simulink model "SF031A_CurrReasbnDiagc"  (R2013b)
settings: Solver=FixedStepDiscrete  SolverMode=SingleTasking  StartTime=0.0  StopTime=1  FixedStep=0.000125  RelTol=1e-3
values from neighbouring files (symbols this model uses):
  ARCHGLBPRM_2MILLISEC_SEC_F32 = DataDict.Constant    [SF031A_CurrReasbnDiagc_DataDict.m]
  ARCHGLBPRM_2PI_ULS_F32 = DataDict.Constant    [SF031A_CurrReasbnDiagc_DataDict.m]
  CurrReasbnDiagcCurrDiagcMotEnvlpTblMax = DataDict.Calibration    [SF031A_CurrReasbnDiagc_DataDict.m]
  CurrReasbnDiagcCurrDiagcPrimErrThd = DataDict.Calibration    [SF031A_CurrReasbnDiagc_DataDict.m]
  CurrReasbnDiagcCurrDiagcSecdryErrThd = DataDict.Calibration    [SF031A_CurrReasbnDiagc_DataDict.m]
  CurrReasbnDiagcCurrDiagcSecdryTqLimThd = DataDict.Calibration    [SF031A_CurrReasbnDiagc_DataDict.m]
  CurrReasbnDiagcDiagFildLim = DataDict.Calibration    [SF031A_CurrReasbnDiagc_DataDict.m]
  CurrReasbnDiagcDiagVltgLpFilEna = DataDict.Calibration    [SF031A_CurrReasbnDiagc_DataDict.m]
  CurrReasbnDiagcLpFilSca = DataDict.Calibration    [SF031A_CurrReasbnDiagc_DataDict.m]
  CurrReasbnDiagcMotVelHiLim = DataDict.Calibration    [SF031A_CurrReasbnDiagc_DataDict.m]
  CurrReasbnDiagcMotVelLoLim = DataDict.Calibration    [SF031A_CurrReasbnDiagc_DataDict.m]
  CurrReasbnDiagcMotVltgQaxDaxFilEna = DataDict.Calibration    [SF031A_CurrReasbnDiagc_DataDict.m]
  CurrReasbnDiagcVelLpFilEna = DataDict.Calibration    [SF031A_CurrReasbnDiagc_DataDict.m]
  ELECGLBPRM_PWMPERDNOMX2_SEC_F32 = DataDict.ConfigParam    [SF031A_CurrReasbnDiagc_DataDict.m]
  NODEBSTEP_CNT_U16 = DataDict.Constant    [SF031A_CurrReasbnDiagc_DataDict.m]
  OffsErrExcdd = DataDict.NTC    [SF031A_CurrReasbnDiagc_DataDict.m]
  ONE_ULS_F32 = DataDict.Constant    [SF031A_CurrReasbnDiagc_DataDict.m]
  ONEOVERTWO_ULS_F32 = DataDict.Constant    [SF031A_CurrReasbnDiagc_DataDict.m]
  SysGlbPrmMotPoleCnt = DataDict.ImprtdCal    [SF031A_CurrReasbnDiagc_DataDict.m]
  TWO_ULS_F32 = DataDict.Constant    [SF031A_CurrReasbnDiagc_DataDict.m]
undefined symbols (not defined in the file or in its folder): NtcSts1
libraries: Fil x8, simulink x6, NxtrLim x3, NxtrMath x2, NexteerUtilities x1
(part 1 of 2)
settings Model: Creator=SZJ6LD  LastModifiedBy=XZ3VZ1
settings DataIOCC: SaveFormat=Structure
settings DebuggingCC: UnderspecifiedInitializationDetection=Simplified  MultiTaskDSMMsg=none

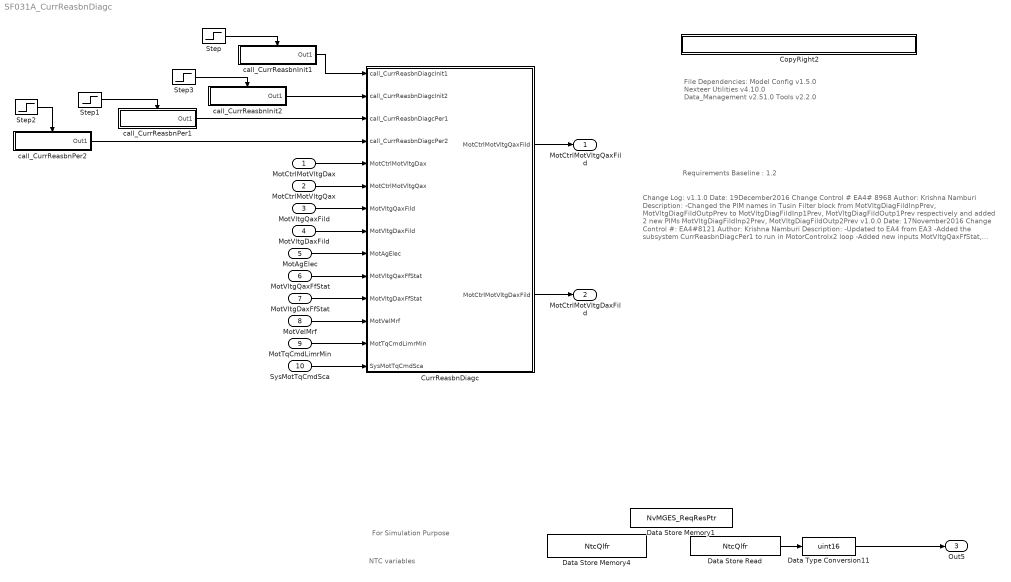
== system SF031A_CurrReasbnDiagc ==
  note: Requirements Baseline : 1.2
  note: File Dependencies:
      |
      | Model Config v1.5.0
      | Nexteer Utilities v4.10.0
      | Data_Management v2.51.0
      | Tools v2.2.0
  note: Change Log:
      |
      | v1.1.0
      | Date: 19December2016
      | Change Control # EA4# 8968
      | Author: Krishna Namburi
      | Description:
      | -Changed the PIM names in Tusin Filter block from MotVltgDiagFildInpPrev, MotVltgDiagFildOutpPrev
      | to  MotVltgDiagFildInp1Prev, MotVltgDiagFildOutp1Prev respectively and added 2 new PIMs
      | MotVltgDiagFildInp2Prev, MotVltgDiagFildOutp2Prev
      |
      | v1.0.0
      | Date: 17November2016
      | Change Control #: EA4#8121
      | Author: Krishna Namburi
      | Description:
      | -Updated to EA4 from EA3
      | -Added the subsystem CurrReasbnDiagcPer1 to run in MotorControlx2 loop
      | -Added new inputs MotVltgQaxFfStat, MotVltgDaxFfStat.
      | - Removed inputs MtrCurrQaxFinalRef_Amp_f32, MtrCurrDaxRef_Amp_f32,EstKe_VpRadpS_f32
      | EstR_Ohm_f32.
      | -Added new outputs MotCtrlMotVltgQaxFild and MotCtrlMotVltgDaxFild.
      | -Removed outputs MotCurrIdptSig_Cnt_u08
      | -Modified CurrReasbnDiagcPer2 subsystem and CurrReasbn Diagnostic subsystem
  note: For Simulation Purpose
  note: NTC variables
  MotCtrlMotVltgDax : Inport  RequirementInfo={} %GIDa_4d26a9da_0edf_44cc_96b7_6099ab8f4765
  MotCtrlMotVltgQax : Inport  RequirementInfo={} %GIDa_b123e9bc_32a7_4223_a27c_0bbcef9fd6da  Port=2
  MotVltgQaxFild : Inport  RequirementInfo={} %GIDa_1c53ad45_08f1_44a0_80ec_49126e27887e  Port=3
  MotVltgDaxFild : Inport  RequirementInfo={} %GIDa_c9186f2c_0f7b_428f_a1bb_4953a8fb6071  Port=4
  MotAgElec : Inport  RequirementInfo={} %GIDa_1a6fc1e2_263f_4c35_82dc_8d7ad84c14ca  Port=5
  MotVltgQaxFfStat : Inport  RequirementInfo={} %GIDa_f597cf15_84d9_42b9_a8ac_86a604ca58ec  Port=6
  MotVltgDaxFfStat : Inport  RequirementInfo={} %GIDa_437fa6bb_7f66_4ed8_b004_d7df1d456be5  Port=7
  MotVelMrf : Inport  RequirementInfo={} %GIDa_277e3cf7_0a4f_44b2_8f78_f4d7dd669071  Port=8
  MotTqCmdLimrMin : Inport  RequirementInfo={} %GIDa_9d945749_2d47_417b_b7b0_0809e9f72747  Port=9
  SysMotTqCmdSca : Inport  RequirementInfo={} %GIDa_449e895f_222c_4d81_855c_0e9bc98e4ae6  Port=10
  CopyRight2 : Subsystem  Description=|  mask(Copyright Information){none=on}
      | Copyright info block.                                               
      |                                                                     
      | Place copyright information at the top of every subsystem in design.
      mask prompts: none "No parameters"
      mask help: Place copyright information at the top of every subsystem in design.
      mask Display:
      | NxtrConf = 'Nexteer Confidential';
      | 
      | sys = bdroot; %handle for the current model ("system")
      | first = get_param(sys,'Created');
      | if(isempty(first))
      |     first = datestr(now,'yyyy');
      | else
      |     first = first(end-3:end);  %year is last four digits
      | end
      | 
      | last = get_param(sys,'LastModifiedDate');
      | if isempty(last)
      |     last = datestr(now,'yyyy');
      | else
      |     last = last(end-3:end);
      | end
      | 
      | if strcmp(first,last)
      |     fprintf('%s -- Copyright %s Nexteer',NxtrConf,first)
      | else
      |     fprintf('%s -- %s%s- %s Nexteer',NxtrConf,char(169),first,last)
      | end
  CurrReasbnDiagc : Subsystem
  Data Store Memory1 : DataStoreMemory  DataStoreName=NvMGES_ReqResPtr  OutDataTypeStr=uint8
  Data Store Read : DataStoreRead  DataStoreName=NtcQlfr  SampleTime=0.1
  Data Store Memory4 : DataStoreMemory  DataStoreName=NtcQlfr  InitialValue=SigQlfr1.SIGQLFR_NORES  OutDataTypeStr=Enum: SigQlfr1
  Data Type Conversion11 : DataTypeConversion  OutDataTypeStr=uint16
  Step : Step  Before=1  After=0  SampleTime=0.000125
  Step1 : Step  SampleTime=0.000125
  Step2 : Step  SampleTime=0.002
  Step3 : Step  Before=1  After=0  SampleTime=0.002
  call_CurrReasbnInit1 : Subsystem  TreatAsAtomicUnit=on
  call_CurrReasbnInit2 : Subsystem  TreatAsAtomicUnit=on
  call_CurrReasbnPer1 : Subsystem  TreatAsAtomicUnit=on
  call_CurrReasbnPer2 : Subsystem  TreatAsAtomicUnit=on
  MotCtrlMotVltgQaxFild : Outport
  MotCtrlMotVltgDaxFild : Outport  Port=2
  Out5 : Outport  Port=3
  wires:
  MotCtrlMotVltgDax/1 -> CurrReasbnDiagc/5(MotCtrlMotVltgDax)
  MotVelMrf/1 -> CurrReasbnDiagc/12(MotVelMrf)
  MotTqCmdLimrMin/1 -> CurrReasbnDiagc/13(MotTqCmdLimrMin)
  SysMotTqCmdSca/1 -> CurrReasbnDiagc/14(SysMotTqCmdSca)
  call_CurrReasbnPer2/1(Out1) -> CurrReasbnDiagc/4(call_CurrReasbnDiagcPer2)
  Step/1 -> call_CurrReasbnInit1/Enable
  Step2/1 -> call_CurrReasbnPer2/Enable
  call_CurrReasbnInit1/1(Out1) -> CurrReasbnDiagc/1(call_CurrReasbnDiagcInit1)
  call_CurrReasbnPer1/1(Out1) -> CurrReasbnDiagc/3(call_CurrReasbnDiagcPer1)
  MotVltgDaxFfStat/1 -> CurrReasbnDiagc/11(MotVltgDaxFfStat)
  MotVltgQaxFfStat/1 -> CurrReasbnDiagc/10(MotVltgQaxFfStat)
  MotAgElec/1 -> CurrReasbnDiagc/9(MotAgElec)
  MotCtrlMotVltgQax/1 -> CurrReasbnDiagc/6(MotCtrlMotVltgQax)
  MotVltgQaxFild/1 -> CurrReasbnDiagc/7(MotVltgQaxFild)
  MotVltgDaxFild/1 -> CurrReasbnDiagc/8(MotVltgDaxFild)
  Step1/1 -> call_CurrReasbnPer1/Enable
  CurrReasbnDiagc/1(MotCtrlMotVltgQaxFild) -> MotCtrlMotVltgQaxFild/1
  CurrReasbnDiagc/2(MotCtrlMotVltgDaxFild) -> MotCtrlMotVltgDaxFild/1
  Data Store Read/1 -> Data Type Conversion11/1
  Data Type Conversion11/1 -> Out5/1
  Step3/1 -> call_CurrReasbnInit2/Enable
  call_CurrReasbnInit2/1(Out1) -> CurrReasbnDiagc/2(call_CurrReasbnDiagcInit2)

== system SF031A_CurrReasbnDiagc/CopyRight2 ==

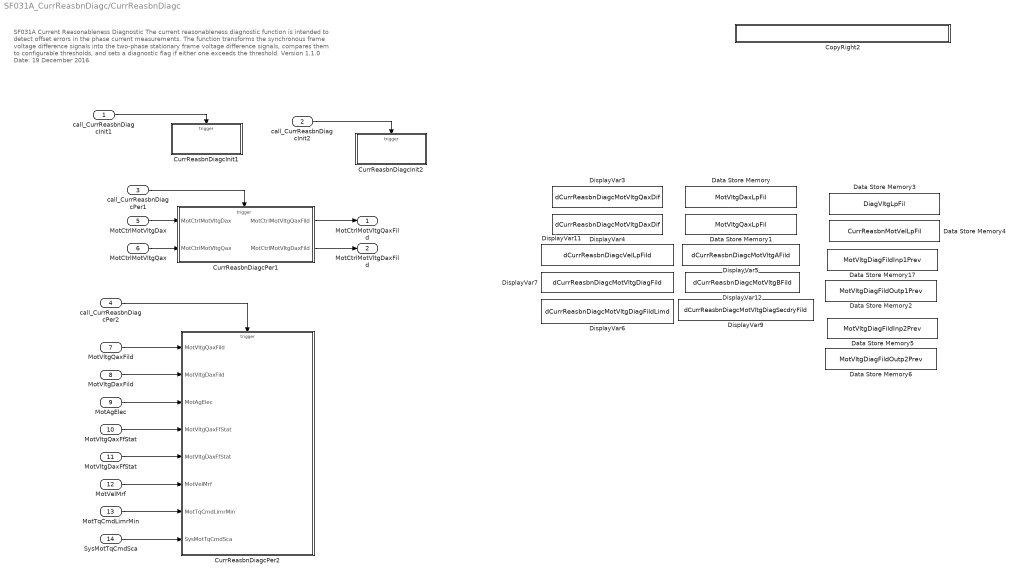
== system SF031A_CurrReasbnDiagc/CurrReasbnDiagc ==
  note: SF031A Current Reasonableness Diagnostic
      |
      | The current reasonableness diagnostic function is intended to detect offset errors in the phase current measurements.
      | The function transforms the synchronous frame voltage difference signals into the two-phase stationary frame voltage difference signals,
      | compares them to configurable thresholds, and sets a diagnostic flag if either one exceeds the threshold.
      | Version 1.1.0   						Date: 19 December 2016
  call_CurrReasbnDiagcInit1 : Inport
  call_CurrReasbnDiagcInit2 : Inport  Port=2
  call_CurrReasbnDiagcPer1 : Inport  RequirementInfo={} %GIDa_f76a18cf_877e_4c65_9912_3a0b33b85457  Port=3
  call_CurrReasbnDiagcPer2 : Inport  RequirementInfo={} %GIDa_cd620524_5019_4baf_8954_3888c8ee52e6  Port=4
  MotCtrlMotVltgDax : Inport  RequirementInfo="{'linktype_rmi_doors' '0000a538 (/E-STEER Core/SubSystem Specifications/Application Functions/SF031A Current Reasonableness Diagnostic)' '#SF031A_101' 'true' 'REQ:  SF031A_101' '' } %GIDa_449d6a4b_7542_48a4_994b_5c51cb8953a2"  Port=5
  MotCtrlMotVltgQax : Inport  RequirementInfo="{'linktype_rmi_doors' '0000a538 (/E-STEER Core/SubSystem Specifications/Application Functions/SF031A Current Reasonableness Diagnostic)' '#SF031A_102' 'true' 'REQ:  SF031A_102' '' } %GIDa_a31c9886_c939_4f41_ac5c_04f44dc75ab9"  Port=6
  MotVltgQaxFild : Inport  RequirementInfo="{'linktype_rmi_doors' '0000a538 (/E-STEER Core/SubSystem Specifications/Application Functions/SF031A Current Reasonableness Diagnostic)' '#SF031A_180' 'true' 'REQ:  SF031A_180' '' } %GIDa_58e0e7bc_af85_4941_a339_39c564b14f0e"  Port=7
  MotVltgDaxFild : Inport  RequirementInfo="{'linktype_rmi_doors' '0000a538 (/E-STEER Core/SubSystem Specifications/Application Functions/SF031A Current Reasonableness Diagnostic)' '#SF031A_181' 'true' 'REQ:  SF031A_181' '' } %GIDa_79f235f9_d307_415b_b321_c5cb8a8df617"  Port=8
  MotAgElec : Inport  RequirementInfo="{'linktype_rmi_doors' '0000a538 (/E-STEER Core/SubSystem Specifications/Application Functions/SF031A Current Reasonableness Diagnostic)' '#SF031A_105' 'true' 'REQ:  SF031A_105' '' } %GIDa_d9cd6df8_3f02_4782_98d1_16055f3fe8b2"  Port=9
  MotVltgQaxFfStat : Inport  RequirementInfo="{'linktype_rmi_doors' '0000a538 (/E-STEER Core/SubSystem Specifications/Application Functions/SF031A Current Reasonableness Diagnostic)' '#SF031A_104' 'true' 'REQ:  SF031A_104' '' } %GIDa_abd8e3fa_7b87_4c29_ad4d_b706a14441a8"  Port=10
  MotVltgDaxFfStat : Inport  RequirementInfo="{'linktype_rmi_doors' '0000a538 (/E-STEER Core/SubSystem Specifications/Application Functions/SF031A Current Reasonableness Diagnostic)' '#SF031A_103' 'true' 'REQ:  SF031A_103' '' } %GIDa_fd47e6d3_2ce2_43f3_87fa_49b3cc0c72b9"  Port=11
  MotVelMrf : Inport  RequirementInfo="{'linktype_rmi_doors' '0000a538 (/E-STEER Core/SubSystem Specifications/Application Functions/SF031A Current Reasonableness Diagnostic)' '#SF031A_113' 'true' 'REQ:  SF031A_113' '' } %GIDa_c5440ddd_8457_4693_9dbb_e70183087e81"  Port=12
  MotTqCmdLimrMin : Inport  RequirementInfo="{'linktype_rmi_doors' '0000a538 (/E-STEER Core/SubSystem Specifications/Application Functions/SF031A Current Reasonableness Diagnostic)' '#SF031A_34' 'true' 'REQ:  SF031A_34' '' } %GIDa_c2343a4c_6c51_4dbf_8cb4_7c8b57a50bd8"  Port=13
  SysMotTqCmdSca : Inport  RequirementInfo="{'linktype_rmi_doors' '0000a538 (/E-STEER Core/SubSystem Specifications/Application Functions/SF031A Current Reasonableness Diagnostic)' '#SF031A_32' 'true' 'REQ:  SF031A_32' '' } %GIDa_aa36bb47_abbb_4a1b_9669_fdecfc6ed391"  Port=14
  CopyRight2 : Subsystem  Description=|  mask(Copyright Information){none=on}
      | Copyright info block.                                               
      |                                                                     
      | Place copyright information at the top of every subsystem in design.
      mask prompts: none "No parameters"
      mask help: Place copyright information at the top of every subsystem in design.
      mask Display:
      | NxtrConf = 'Nexteer Confidential';
      | 
      | sys = bdroot; %handle for the current model ("system")
      | first = get_param(sys,'Created');
      | if(isempty(first))
      |     first = datestr(now,'yyyy');
      | else
      |     first = first(end-3:end);  %year is last four digits
      | end
      | 
      | last = get_param(sys,'LastModifiedDate');
      | if isempty(last)
      |     last = datestr(now,'yyyy');
      | else
      |     last = last(end-3:end);
      | end
      | 
      | if strcmp(first,last)
      |     fprintf('%s -- Copyright %s Nexteer',NxtrConf,first)
      | else
      |     fprintf('%s -- %s%s- %s Nexteer',NxtrConf,char(169),first,last)
      | end
  CurrReasbnDiagcInit1 : Subsystem
  CurrReasbnDiagcInit2 : Subsystem
  CurrReasbnDiagcPer1 : Subsystem
  CurrReasbnDiagcPer2 : Subsystem
  Data Store Memory : DataStoreMemory  DataStoreName=MotVltgDaxLpFil  InitialValue=[]  StateMustResolveToSignalObject=on
  Data Store Memory1 : DataStoreMemory  DataStoreName=MotVltgQaxLpFil  InitialValue=[]  StateMustResolveToSignalObject=on
  Data Store Memory17 : DataStoreMemory  DataStoreName=MotVltgDiagFildInp1Prev  StateMustResolveToSignalObject=on
  Data Store Memory2 : DataStoreMemory  DataStoreName=MotVltgDiagFildOutp1Prev  StateMustResolveToSignalObject=on
  Data Store Memory3 : DataStoreMemory  DataStoreName=DiagVltgLpFil  InitialValue=[]  StateMustResolveToSignalObject=on
  Data Store Memory4 : DataStoreMemory  DataStoreName=CurrReasbnMotVelLpFil  InitialValue=[]  StateMustResolveToSignalObject=on
  Data Store Memory5 : DataStoreMemory  DataStoreName=MotVltgDiagFildInp2Prev  StateMustResolveToSignalObject=on
  Data Store Memory6 : DataStoreMemory  DataStoreName=MotVltgDiagFildOutp2Prev  StateMustResolveToSignalObject=on
  DisplayVar11 : DataStoreMemory  DataStoreName=dCurrReasbnDiagcVelLpFild  ReadBeforeWriteMsg=warning  WriteAfterWriteMsg=warning  WriteAfterReadMsg=warning  StateMustResolveToSignalObject=on
  DisplayVar12 : DataStoreMemory  DataStoreName=dCurrReasbnDiagcMotVltgBFild  ReadBeforeWriteMsg=warning  WriteAfterWriteMsg=warning  WriteAfterReadMsg=warning  StateMustResolveToSignalObject=on
  DisplayVar3 : DataStoreMemory  DataStoreName=dCurrReasbnDiagcMotVltgQaxDif  ReadBeforeWriteMsg=warning  WriteAfterWriteMsg=warning  WriteAfterReadMsg=warning  StateMustResolveToSignalObject=on
  DisplayVar4 : DataStoreMemory  DataStoreName=dCurrReasbnDiagcMotVltgDaxDif  ReadBeforeWriteMsg=warning  WriteAfterWriteMsg=warning  WriteAfterReadMsg=warning  StateMustResolveToSignalObject=on
  DisplayVar5 : DataStoreMemory  DataStoreName=dCurrReasbnDiagcMotVltgAFild  ReadBeforeWriteMsg=warning  WriteAfterWriteMsg=warning  WriteAfterReadMsg=warning  StateMustResolveToSignalObject=on
  DisplayVar6 : DataStoreMemory  DataStoreName=dCurrReasbnDiagcMotVltgDiagFildLimd  ReadBeforeWriteMsg=warning  WriteAfterWriteMsg=warning  WriteAfterReadMsg=warning  StateMustResolveToSignalObject=on
  DisplayVar7 : DataStoreMemory  DataStoreName=dCurrReasbnDiagcMotVltgDiagFild  ReadBeforeWriteMsg=warning  WriteAfterWriteMsg=warning  WriteAfterReadMsg=warning  StateMustResolveToSignalObject=on
  DisplayVar9 : DataStoreMemory  DataStoreName=dCurrReasbnDiagcMotVltgDiagSecdryFild  ReadBeforeWriteMsg=warning  WriteAfterWriteMsg=warning  WriteAfterReadMsg=warning  StateMustResolveToSignalObject=on
  MotCtrlMotVltgQaxFild : Outport  RequirementInfo="{'linktype_rmi_doors' '0000a538 (/E-STEER Core/SubSystem Specifications/Application Functions/SF031A Current Reasonableness Diagnostic)' '#SF031A_183' 'true' 'REQ:  SF031A_183' '' ; 'linktype_rmi_doors' '0000a538 (/E-STEER Core/SubSystem Specifications/Application Functions/SF031A Current Reasonableness Diagnostic)' '#SF031A_53' 'true' 'REQ:  SF031A_53' '' } %GIDa_ce180fd6_f185_48df_8933_7de0682d2221"
  MotCtrlMotVltgDaxFild : Outport  RequirementInfo="{'linktype_rmi_doors' '0000a538 (/E-STEER Core/SubSystem Specifications/Application Functions/SF031A Current Reasonableness Diagnostic)' '#SF031A_184' 'true' 'REQ:  SF031A_184' '' ; 'linktype_rmi_doors' '0000a538 (/E-STEER Core/SubSystem Specifications/Application Functions/SF031A Current Reasonableness Diagnostic)' '#SF031A_188' 'true' 'REQ:  SF031A_188' '' } %GIDa_5c3c9398_cb08_40a3_88f4_91205b1bad21"  Port=2
  wires:
  MotCtrlMotVltgDax/1 -> CurrReasbnDiagcPer1/1(MotCtrlMotVltgDax)
  MotCtrlMotVltgQax/1 -> CurrReasbnDiagcPer1/2(MotCtrlMotVltgQax)
  MotAgElec/1 -> CurrReasbnDiagcPer2/3(MotAgElec)
  MotVltgQaxFfStat/1 -> CurrReasbnDiagcPer2/4(MotVltgQaxFfStat)
  MotVltgDaxFfStat/1 -> CurrReasbnDiagcPer2/5(MotVltgDaxFfStat)
  MotVelMrf/1 -> CurrReasbnDiagcPer2/6(MotVelMrf)
  MotTqCmdLimrMin/1 -> CurrReasbnDiagcPer2/7(MotTqCmdLimrMin)
  SysMotTqCmdSca/1 -> CurrReasbnDiagcPer2/8(SysMotTqCmdSca)
  call_CurrReasbnDiagcInit1/1 -> CurrReasbnDiagcInit1/Trigger
  call_CurrReasbnDiagcPer1/1 -> CurrReasbnDiagcPer1/Trigger
  call_CurrReasbnDiagcPer2/1 -> CurrReasbnDiagcPer2/Trigger
  CurrReasbnDiagcPer1/1(MotCtrlMotVltgQaxFild) -> MotCtrlMotVltgQaxFild/1
  CurrReasbnDiagcPer1/2(MotCtrlMotVltgDaxFild) -> MotCtrlMotVltgDaxFild/1
  MotVltgQaxFild/1 -> CurrReasbnDiagcPer2/1(MotVltgQaxFild)
  MotVltgDaxFild/1 -> CurrReasbnDiagcPer2/2(MotVltgDaxFild)
  call_CurrReasbnDiagcInit2/1 -> CurrReasbnDiagcInit2/Trigger

== system SF031A_CurrReasbnDiagc/call_CurrReasbnInit1 ==
  Enable : EnablePort
  Function-Call Generator : simulink/Ports & Subsystems/Function-Call Generator  sample_time=0.000125  numberOfIterations=1
  Out1 : Outport
  wires:
  Function-Call Generator/1 -> Out1/1

== system SF031A_CurrReasbnDiagc/call_CurrReasbnInit2 ==
  Enable : EnablePort
  Function-Call Generator : simulink/Ports & Subsystems/Function-Call Generator  sample_time=0.002  numberOfIterations=1
  Out1 : Outport
  wires:
  Function-Call Generator/1 -> Out1/1

== system SF031A_CurrReasbnDiagc/call_CurrReasbnPer1 ==
  Enable : EnablePort
  Function-Call Generator : simulink/Ports & Subsystems/Function-Call Generator  sample_time=0.002  numberOfIterations=1
  Out1 : Outport
  wires:
  Function-Call Generator/1 -> Out1/1

== system SF031A_CurrReasbnDiagc/call_CurrReasbnPer2 ==
  Enable : EnablePort
  Function-Call Generator : simulink/Ports & Subsystems/Function-Call Generator  sample_time=0.1  numberOfIterations=1
  Out1 : Outport
  wires:
  Function-Call Generator/1 -> Out1/1

== system SF031A_CurrReasbnDiagc/CurrReasbnDiagc/CopyRight2 ==

== system SF031A_CurrReasbnDiagc/CurrReasbnDiagc/CurrReasbnDiagcInit1 ==
  Function : TriggerPort  TriggerType=function-call  PortDimensions=1
  CopyRight2 : Subsystem  Description=|  mask(Copyright Information){none=on}
      | Copyright info block.                                               
      |                                                                     
      | Place copyright information at the top of every subsystem in design.
      mask prompts: none "No parameters"
      mask help: Place copyright information at the top of every subsystem in design.
      mask Display:
      | NxtrConf = 'Nexteer Confidential';
      | 
      | sys = bdroot; %handle for the current model ("system")
      | first = get_param(sys,'Created');
      | if(isempty(first))
      |     first = datestr(now,'yyyy');
      | else
      |     first = first(end-3:end);  %year is last four digits
      | end
      | 
      | last = get_param(sys,'LastModifiedDate');
      | if isempty(last)
      |     last = datestr(now,'yyyy');
      | else
      |     last = last(end-3:end);
      | end
      | 
      | if strcmp(first,last)
      |     fprintf('%s -- Copyright %s Nexteer',NxtrConf,first)
      | else
      |     fprintf('%s -- %s%s- %s Nexteer',NxtrConf,char(169),first,last)
      | end
  MotVltgDaxLpFil : Fil/FilLpInit  RequirementInfo="{'linktype_rmi_doors' '0000a538 (/E-STEER Core/SubSystem Specifications/Application Functions/SF031A Current Reasonableness Diagnostic)' '#SF031A_117' 'true' 'REQ:  SF031A_117' '' ; 'linktype_rmi_doors' '0000a538 (/E-STEER Core/SubSystem Specifications/Application Functions/SF031A Current Reasonableness Diagnostic)' '#SF031A_118' 'true' 'REQ:  SF031A_118' '' ; 'linktype_rmi_doors' '0000a538 (/E-STEER Core/SubSystem Specifications/Application Functions/SF031A Current Reasonableness Diagnostic)' '#SF031A_119' 'true' 'REQ:  SF031A_119' '' } %GIDa_545bb3fc_f7bc_47c5_a864_b622a625ba7e"  Ic=0  Ts=ELECGLBPRM_PWMPERDNOMX2_SEC_F32  Freq=CurrReasbnDiagcMotVltgDaxLpFilFrq  StVar=MotVltgDaxLpFil
  MotVltgQaxLpFil : Fil/FilLpInit  RequirementInfo="{'linktype_rmi_doors' '0000a538 (/E-STEER Core/SubSystem Specifications/Application Functions/SF031A Current Reasonableness Diagnostic)' '#SF031A_120' 'true' 'REQ:  SF031A_120' '' ; 'linktype_rmi_doors' '0000a538 (/E-STEER Core/SubSystem Specifications/Application Functions/SF031A Current Reasonableness Diagnostic)' '#SF031A_121' 'true' 'REQ:  SF031A_121' '' ; 'linktype_rmi_doors' '0000a538 (/E-STEER Core/SubSystem Specifications/Application Functions/SF031A Current Reasonableness Diagnostic)' '#SF031A_122' 'true' 'REQ:  SF031A_122' '' } %GIDa_604bee18_9ac3_4a74_b746_90fd54a7749f"  Ic=0  Ts=ELECGLBPRM_PWMPERDNOMX2_SEC_F32  Freq=CurrReasbnDiagcMotVltgQaxLpFilFrq  StVar=MotVltgQaxLpFil

== system SF031A_CurrReasbnDiagc/CurrReasbnDiagc/CurrReasbnDiagcInit2 ==
  Function : TriggerPort  TriggerType=function-call  PortDimensions=1
  CopyRight2 : Subsystem  Description=|  mask(Copyright Information){none=on}
      | Copyright info block.                                               
      |                                                                     
      | Place copyright information at the top of every subsystem in design.
      mask prompts: none "No parameters"
      mask help: Place copyright information at the top of every subsystem in design.
      mask Display:
      | NxtrConf = 'Nexteer Confidential';
      | 
      | sys = bdroot; %handle for the current model ("system")
      | first = get_param(sys,'Created');
      | if(isempty(first))
      |     first = datestr(now,'yyyy');
      | else
      |     first = first(end-3:end);  %year is last four digits
      | end
      | 
      | last = get_param(sys,'LastModifiedDate');
      | if isempty(last)
      |     last = datestr(now,'yyyy');
      | else
      |     last = last(end-3:end);
      | end
      | 
      | if strcmp(first,last)
      |     fprintf('%s -- Copyright %s Nexteer',NxtrConf,first)
      | else
      |     fprintf('%s -- %s%s- %s Nexteer',NxtrConf,char(169),first,last)
      | end
  DiagVltgLpFil : Fil/FilLpInit  RequirementInfo="{'linktype_rmi_doors' '0000a538 (/E-STEER Core/SubSystem Specifications/Application Functions/SF031A Current Reasonableness Diagnostic)' '#SF031A_55' 'true' 'REQ:  SF031A_55' '' ; 'linktype_rmi_doors' '0000a538 (/E-STEER Core/SubSystem Specifications/Application Functions/SF031A Current Reasonableness Diagnostic)' '#SF031A_68' 'true' 'REQ:  SF031A_68' '' ; 'linktype_rmi_doors' '0000a538 (/E-STEER Core/SubSystem Specifications/Application Functions/SF031A Current Reasonableness Diagnostic)' '#SF031A_69' 'true' 'REQ:  SF031A_69' '' } %GIDa_a4e20848_ba57_4acb_8d1e_03c55eb94fa5"  Ic=0  Ts=ARCHGLBPRM_2MILLISEC_SEC_F32  Freq=CurrReasbnDiagcDiagVltgLpFilFrq  StVar=DiagVltgLpFil
  MotVelLpFil : Fil/FilLpInit  RequirementInfo="{'linktype_rmi_doors' '0000a538 (/E-STEER Core/SubSystem Specifications/Application Functions/SF031A Current Reasonableness Diagnostic)' '#SF031A_135' 'true' 'REQ:  SF031A_135' '' ; 'linktype_rmi_doors' '0000a538 (/E-STEER Core/SubSystem Specifications/Application Functions/SF031A Current Reasonableness Diagnostic)' '#SF031A_136' 'true' 'REQ:  SF031A_136' '' ; 'linktype_rmi_doors' '0000a538 (/E-STEER Core/SubSystem Specifications/Application Functions/SF031A Current Reasonableness Diagnostic)' '#SF031A_137' 'true' 'REQ:  SF031A_137' '' } %GIDa_38e4ad57_fc16_456c_8108_9d804f014d91"  Ic=0  Ts=ARCHGLBPRM_2MILLISEC_SEC_F32  Freq=CurrReasbnDiagcVelLpFilFrq  StVar=CurrReasbnMotVelLpFil

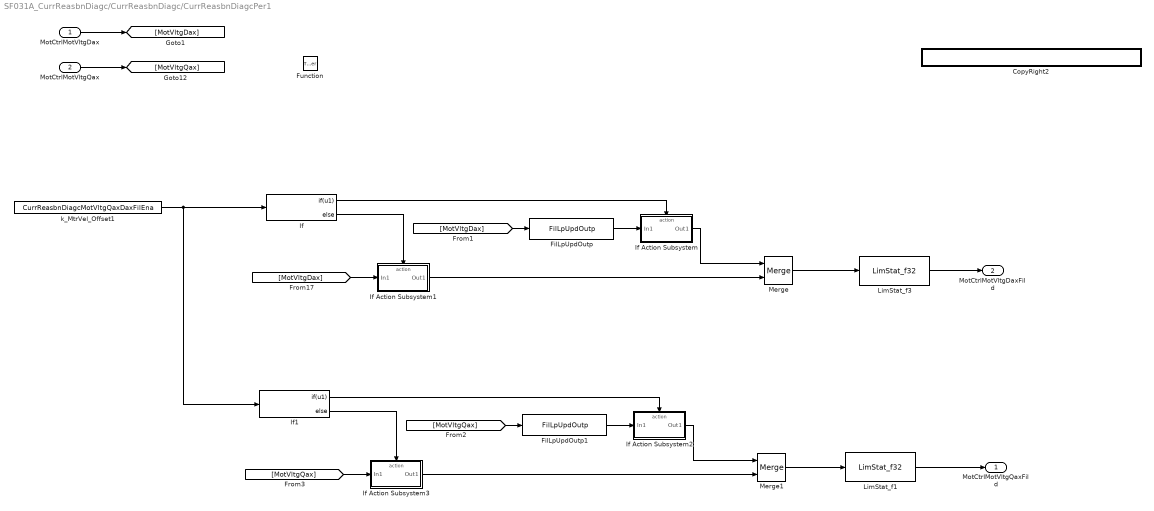
== system SF031A_CurrReasbnDiagc/CurrReasbnDiagc/CurrReasbnDiagcPer1 ==
  MotCtrlMotVltgDax : Inport
  MotCtrlMotVltgQax : Inport  Port=2
  Function : TriggerPort  TriggerType=function-call  PortDimensions=1
  CopyRight2 : Subsystem  Description=|  mask(Copyright Information){none=on}
      | Copyright info block.                                               
      |                                                                     
      | Place copyright information at the top of every subsystem in design.
      mask prompts: none "No parameters"
      mask help: Place copyright information at the top of every subsystem in design.
      mask Display:
      | NxtrConf = 'Nexteer Confidential';
      | 
      | sys = bdroot; %handle for the current model ("system")
      | first = get_param(sys,'Created');
      | if(isempty(first))
      |     first = datestr(now,'yyyy');
      | else
      |     first = first(end-3:end);  %year is last four digits
      | end
      | 
      | last = get_param(sys,'LastModifiedDate');
      | if isempty(last)
      |     last = datestr(now,'yyyy');
      | else
      |     last = last(end-3:end);
      | end
      | 
      | if strcmp(first,last)
      |     fprintf('%s -- Copyright %s Nexteer',NxtrConf,first)
      | else
      |     fprintf('%s -- %s%s- %s Nexteer',NxtrConf,char(169),first,last)
      | end
  FilLpUpdOutp : Fil/FilLpUpdOutp  RequirementInfo="{'linktype_rmi_doors' '0000a538 (/E-STEER Core/SubSystem Specifications/Application Functions/SF031A Current Reasonableness Diagnostic)' '#SF031A_119' 'true' 'REQ:  SF031A_119' '' } %GIDa_0bdcd772_3d94_4ed3_9d8e_9a962b62be66"  StVar=MotVltgDaxLpFil
      settings: AttributesFormatString=StVar: %<StVar>
  FilLpUpdOutp1 : Fil/FilLpUpdOutp  RequirementInfo="{'linktype_rmi_doors' '0000a538 (/E-STEER Core/SubSystem Specifications/Application Functions/SF031A Current Reasonableness Diagnostic)' '#SF031A_122' 'true' 'REQ:  SF031A_122' '' } %GIDa_c6ec76a7_5629_4356_a502_1eddb003cac3"  StVar=MotVltgQaxLpFil
      settings: AttributesFormatString=StVar: %<StVar>
  If : If  RequirementInfo={} %GIDa_4eaed197_11a7_40f2_86a5_1975bdcb76d0  IfExpression=u1
  If Action Subsystem : Subsystem  RequirementInfo={} %GIDa_00c2fa5a_fbc3_441c_a367_37dfae2dbef4  TreatAsAtomicUnit=on
  If Action Subsystem1 : Subsystem  RequirementInfo="{'linktype_rmi_doors' '0000a538 (/E-STEER Core/SubSystem Specifications/Application Functions/SF031A Current Reasonableness Diagnostic)' '#SF031A_128' 'true' 'REQ:  SF031A_128' '' } %GIDa_1fe47eb7_a113_469c_ad99_cc162c2c38d6"  TreatAsAtomicUnit=on
  If Action Subsystem2 : Subsystem  RequirementInfo={} %GIDa_c58246ad_3913_453b_9486_f2482565a650  TreatAsAtomicUnit=on
  If Action Subsystem3 : Subsystem  RequirementInfo="{'linktype_rmi_doors' '0000a538 (/E-STEER Core/SubSystem Specifications/Application Functions/SF031A Current Reasonableness Diagnostic)' '#SF031A_128' 'true' 'REQ:  SF031A_128' '' } %GIDa_31ccc5af_544e_445b_9515_48ac232701ab"  TreatAsAtomicUnit=on
  If1 : If  RequirementInfo={} %GIDa_aaf01723_13a8_4e1a_9d66_cdf0fa002415  IfExpression=u1
  LimStat_f1 : NxtrLim/LimStat_f32  RequirementInfo="{'linktype_rmi_doors' '0000a538 (/E-STEER Core/SubSystem Specifications/Application Functions/SF031A Current Reasonableness Diagnostic)' '#SF031A_54' 'true' 'REQ:  SF031A_54' '' } %GIDa_91209a5f_9287_41d6_91f8_6493ea078b8b"  LoLim=MOTVLTGFILDDQAXLOLIM_VOLT_F32  HiLim=MOTVLTGFILDDQAXHILIM_VOLT_F32
      settings: AttributesFormatString=|
      | Low Limit: %<LoLim>
      | High Limit:%<HiLim>
  LimStat_f3 : NxtrLim/LimStat_f32  RequirementInfo="{'linktype_rmi_doors' '0000a538 (/E-STEER Core/SubSystem Specifications/Application Functions/SF031A Current Reasonableness Diagnostic)' '#SF031A_54' 'true' 'REQ:  SF031A_54' '' } %GIDa_4d541c39_a59f_4acb_bc66_4e759b09bfe0"  LoLim=MOTVLTGFILDDQAXLOLIM_VOLT_F32  HiLim=MOTVLTGFILDDQAXHILIM_VOLT_F32
      settings: AttributesFormatString=|
      | Low Limit: %<LoLim>
      | High Limit:%<HiLim>
  Merge : Merge  RequirementInfo={} %GIDa_fb066bc8_6024_4dde_9dee_e34aae3272bf
  Merge1 : Merge  RequirementInfo={} %GIDa_7cbaeab9_1e18_469d_af75_bf02b1206196
  k_MtrVel_Offset1 : Constant  RequirementInfo="{'linktype_rmi_doors' '0000a538 (/E-STEER Core/SubSystem Specifications/Application Functions/SF031A Current Reasonableness Diagnostic)' '#SF031A_123' 'true' 'REQ:  SF031A_123' '' ; 'linktype_rmi_doors' '0000a538 (/E-STEER Core/SubSystem Specifications/Application Functions/SF031A Current Reasonableness Diagnostic)' '#SF031A_125' 'true' 'REQ:  SF031A_125' '' ; 'linktype_rmi_doors' '0000a538 (/E-STEER Core/SubSystem Specifications/Application Functions/SF031A Current Reasonableness Diagnostic)' '#SF031A_126' 'true' 'REQ:  SF031A_126' '' } %GIDa_e297f351_dc06_46c0_a820_c79be0c6f900"  Value=CurrReasbnDiagcMotVltgQaxDaxFilEna
  MotCtrlMotVltgQaxFild : Outport  RequirementInfo="{'linktype_rmi_doors' '0000a538 (/E-STEER Core/SubSystem Specifications/Application Functions/SF031A Current Reasonableness Diagnostic)' '#SF031A_116' 'true' 'REQ:  SF031A_116' '' } %GIDa_45e1c268_1e65_407c_afe4_4fc7519d281d"
  MotCtrlMotVltgDaxFild : Outport  RequirementInfo="{'linktype_rmi_doors' '0000a538 (/E-STEER Core/SubSystem Specifications/Application Functions/SF031A Current Reasonableness Diagnostic)' '#SF031A_115' 'true' 'REQ:  SF031A_115' '' } %GIDa_c27bf963_d5b6_4a40_a2f0_af90b46b3739"  Port=2
  wires:
  If/2 -> If Action Subsystem1/Action
  If/1 -> If Action Subsystem/Action
  If Action Subsystem/1(Out1) -> Merge/1
  If Action Subsystem1/1(Out1) -> Merge/2
  FilLpUpdOutp/1 -> If Action Subsystem/1(In1)
  MotCtrlMotVltgQax/1 -> [MotVltgQax]
  MotCtrlMotVltgDax/1 -> [MotVltgDax]
  [MotVltgDax] -> If Action Subsystem1/1(In1)
  [MotVltgDax] -> FilLpUpdOutp/1
  k_MtrVel_Offset1/1 -> If1/1, If/1
  If1/2 -> If Action Subsystem3/Action
  If1/1 -> If Action Subsystem2/Action
  If Action Subsystem2/1(Out1) -> Merge1/1
  If Action Subsystem3/1(Out1) -> Merge1/2
  FilLpUpdOutp1/1 -> If Action Subsystem2/1(In1)
  [MotVltgQax] -> If Action Subsystem3/1(In1)
  [MotVltgQax] -> FilLpUpdOutp1/1
  Merge1/1 -> LimStat_f1/1
  Merge/1 -> LimStat_f3/1
  LimStat_f3/1 -> MotCtrlMotVltgDaxFild/1
  LimStat_f1/1 -> MotCtrlMotVltgQaxFild/1

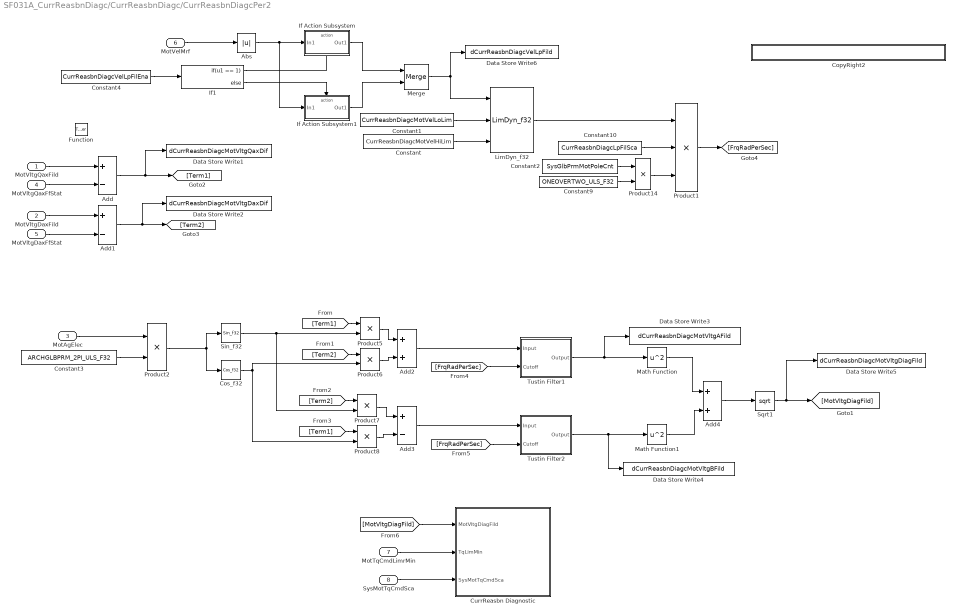
== system SF031A_CurrReasbnDiagc/CurrReasbnDiagc/CurrReasbnDiagcPer2 ==
  MotVltgQaxFild : Inport
  MotVltgDaxFild : Inport  Port=2
  MotAgElec : Inport  RequirementInfo="{'linktype_rmi_doors' '0000a538 (/E-STEER Core/SubSystem Specifications/Application Functions/SF031A Current Reasonableness Diagnostic)' '#SF031A_111' 'true' 'REQ:  SF031A_111' '' } %GIDa_bb017c90_8ba2_4a6e_b20d_7995ad9382d5"  Port=3
  MotVltgQaxFfStat : Inport  Port=4
  MotVltgDaxFfStat : Inport  Port=5
  MotVelMrf : Inport  RequirementInfo="{'linktype_rmi_doors' '0000a538 (/E-STEER Core/SubSystem Specifications/Application Functions/SF031A Current Reasonableness Diagnostic)' '#SF031A_161' 'true' 'REQ:  SF031A_161' '' } %GIDa_967b09cf_1cb4_48cc_97c8_cfe5406b841b"  Port=6
  MotTqCmdLimrMin : Inport  Port=7
  SysMotTqCmdSca : Inport  Port=8
  Function : TriggerPort  TriggerType=function-call  PortDimensions=1
  Abs : Abs  RequirementInfo="{'linktype_rmi_doors' '0000a538 (/E-STEER Core/SubSystem Specifications/Application Functions/SF031A Current Reasonableness Diagnostic)' '#SF031A_161' 'true' 'REQ:  SF031A_161' '' } %GIDa_d54369ce_abbe_4764_970b_c7cf26a8a4e7"
  Add : Sum  RequirementInfo="{'linktype_rmi_doors' '0000a538 (/E-STEER Core/SubSystem Specifications/Application Functions/SF031A Current Reasonableness Diagnostic)' '#SF031A_110' 'true' 'REQ:  SF031A_110' '' } %GIDa_43892b87_f712_4b65_87f1_f9f131bc7353"  Inputs=+-
  Add1 : Sum  RequirementInfo="{'linktype_rmi_doors' '0000a538 (/E-STEER Core/SubSystem Specifications/Application Functions/SF031A Current Reasonableness Diagnostic)' '#SF031A_109' 'true' 'REQ:  SF031A_109' '' } %GIDa_58d41568_c7f8_422c_ab01_217b8c371e9b"  Inputs=+-
  Add2 : Sum  RequirementInfo="{'linktype_rmi_doors' '0000a538 (/E-STEER Core/SubSystem Specifications/Application Functions/SF031A Current Reasonableness Diagnostic)' '#SF031A_111' 'true' 'REQ:  SF031A_111' '' } %GIDa_3a30e3e6_d748_43f6_bde7_757f7a0c2edf"
  Add3 : Sum  RequirementInfo="{'linktype_rmi_doors' '0000a538 (/E-STEER Core/SubSystem Specifications/Application Functions/SF031A Current Reasonableness Diagnostic)' '#SF031A_112' 'true' 'REQ:  SF031A_112' '' } %GIDa_b628f4b1_0a20_4162_abd2_5e1597dd7059"  Inputs=+-
  Add4 : Sum  RequirementInfo="{'linktype_rmi_doors' '0000a538 (/E-STEER Core/SubSystem Specifications/Application Functions/SF031A Current Reasonableness Diagnostic)' '#SF031A_159' 'true' 'REQ:  SF031A_159' '' } %GIDa_960b96c1_6ca7_4020_ad57_9fe81e91346a"
  Constant : Constant  RequirementInfo="{'linktype_rmi_doors' '0000a538 (/E-STEER Core/SubSystem Specifications/Application Functions/SF031A Current Reasonableness Diagnostic)' '#SF031A_143' 'true' 'REQ:  SF031A_143' '' ; 'linktype_rmi_doors' '0000a538 (/E-STEER Core/SubSystem Specifications/Application Functions/SF031A Current Reasonableness Diagnostic)' '#SF031A_144' 'true' 'REQ:  SF031A_144' '' ; 'linktype_rmi_doors' '0000a538 (/E-STEER Core/SubSystem Specifications/Application Functions/SF031A Current Reasonableness Diagnostic)' '#SF031A_145' 'true' 'REQ:  SF031A_145' '' } %GIDa_a5e1b34e_9da0_4e67_bef9_6fcb770a7617"  Value=CurrReasbnDiagcMotVelHiLim
  Constant1 : Constant  RequirementInfo="{'linktype_rmi_doors' '0000a538 (/E-STEER Core/SubSystem Specifications/Application Functions/SF031A Current Reasonableness Diagnostic)' '#SF031A_140' 'true' 'REQ:  SF031A_140' '' ; 'linktype_rmi_doors' '0000a538 (/E-STEER Core/SubSystem Specifications/Application Functions/SF031A Current Reasonableness Diagnostic)' '#SF031A_141' 'true' 'REQ:  SF031A_141' '' ; 'linktype_rmi_doors' '0000a538 (/E-STEER Core/SubSystem Specifications/Application Functions/SF031A Current Reasonableness Diagnostic)' '#SF031A_142' 'true' 'REQ:  SF031A_142' '' } %GIDa_3e3e03f2_ebf0_403a_b88a_becb6acf790f"  Value=CurrReasbnDiagcMotVelLoLim
  Constant10 : Constant  RequirementInfo="{'linktype_rmi_doors' '0000a538 (/E-STEER Core/SubSystem Specifications/Application Functions/SF031A Current Reasonableness Diagnostic)' '#SF031A_148' 'true' 'REQ:  SF031A_148' '' ; 'linktype_rmi_doors' '0000a538 (/E-STEER Core/SubSystem Specifications/Application Functions/SF031A Current Reasonableness Diagnostic)' '#SF031A_149' 'true' 'REQ:  SF031A_149' '' ; 'linktype_rmi_doors' '0000a538 (/E-STEER Core/SubSystem Specifications/Application Functions/SF031A Current Reasonableness Diagnostic)' '#SF031A_150' 'true' 'REQ:  SF031A_150' '' } %GIDa_f6e31673_0347_40ee_8ad4_3df059a66b96"  Value=CurrReasbnDiagcLpFilSca
  Constant2 : Constant  Value=SysGlbPrmMotPoleCnt
  Constant3 : Constant  RequirementInfo="{'linktype_rmi_doors' '0000a538 (/E-STEER Core/SubSystem Specifications/Application Functions/SF031A Current Reasonableness Diagnostic)' '#SF031A_111' 'true' 'REQ:  SF031A_111' '' } %GIDa_75513eea_adac_4531_a3e9_6d937e917c0d"  Value=ARCHGLBPRM_2PI_ULS_F32
  Constant4 : Constant  RequirementInfo="{'linktype_rmi_doors' '0000a538 (/E-STEER Core/SubSystem Specifications/Application Functions/SF031A Current Reasonableness Diagnostic)' '#SF031A_131' 'true' 'REQ:  SF031A_131' '' ; 'linktype_rmi_doors' '0000a538 (/E-STEER Core/SubSystem Specifications/Application Functions/SF031A Current Reasonableness Diagnostic)' '#SF031A_132' 'true' 'REQ:  SF031A_132' '' ; 'linktype_rmi_doors' '0000a538 (/E-STEER Core/SubSystem Specifications/Application Functions/SF031A Current Reasonableness Diagnostic)' '#SF031A_133' 'true' 'REQ:  SF031A_133' '' } %GIDa_45d72eda_53f7_4f3b_9665_a622aad47224"  Value=CurrReasbnDiagcVelLpFilEna
  Constant9 : Constant  Value=ONEOVERTWO_ULS_F32
  CopyRight2 : Subsystem  Description=|  mask(Copyright Information){none=on}
      | Copyright info block.                                               
      |                                                                     
      | Place copyright information at the top of every subsystem in design.
      mask prompts: none "No parameters"
      mask help: Place copyright information at the top of every subsystem in design.
      mask Display:
      | NxtrConf = 'Nexteer Confidential';
      | 
      | sys = bdroot; %handle for the current model ("system")
      | first = get_param(sys,'Created');
      | if(isempty(first))
      |     first = datestr(now,'yyyy');
      | else
      |     first = first(end-3:end);  %year is last four digits
      | end
      | 
      | last = get_param(sys,'LastModifiedDate');
      | if isempty(last)
      |     last = datestr(now,'yyyy');
      | else
      |     last = last(end-3:end);
      | end
      | 
      | if strcmp(first,last)
      |     fprintf('%s -- Copyright %s Nexteer',NxtrConf,first)
      | else
      |     fprintf('%s -- %s%s- %s Nexteer',NxtrConf,char(169),first,last)
      | end
  Cos_f32 : NxtrMath/Cos_f32  SFunctionSpec=single y1 = Cos_f32(single u1)
      settings: AttributesFormatString=%<MaskType>
  CurrReasbn Diagnostic : Subsystem
  Data Store Write1 : DataStoreWrite  DataStoreName=dCurrReasbnDiagcMotVltgQaxDif
  Data Store Write2 : DataStoreWrite  DataStoreName=dCurrReasbnDiagcMotVltgDaxDif
  Data Store Write3 : DataStoreWrite  RequirementInfo="{'linktype_rmi_doors' '0000a538 (/E-STEER Core/SubSystem Specifications/Application Functions/SF031A Current Reasonableness Diagnostic)' '#SF031A_159' 'true' 'REQ:  SF031A_159' '' } %GIDa_08206768_f0eb_46ac_9e16_71ad0fcb94c3"  DataStoreName=dCurrReasbnDiagcMotVltgAFild
  Data Store Write4 : DataStoreWrite  DataStoreName=dCurrReasbnDiagcMotVltgBFild
  Data Store Write5 : DataStoreWrite  RequirementInfo="{'linktype_rmi_doors' '0000a538 (/E-STEER Core/SubSystem Specifications/Application Functions/SF031A Current Reasonableness Diagnostic)' '#SF031A_159' 'true' 'REQ:  SF031A_159' '' } %GIDa_d960d700_bb3f_412c_bd6c_9ef7dae987b4"  DataStoreName=dCurrReasbnDiagcMotVltgDiagFild
  Data Store Write6 : DataStoreWrite  DataStoreName=dCurrReasbnDiagcVelLpFild
  If Action Subsystem : Subsystem  RequirementInfo="{'linktype_rmi_doors' '0000a538 (/E-STEER Core/SubSystem Specifications/Application Functions/SF031A Current Reasonableness Diagnostic)' '#SF031A_134' 'true' 'REQ:  SF031A_134' '' } %GIDa_e494de51_55d9_49e8_8e8f_5416ff53702d"  TreatAsAtomicUnit=on
  If Action Subsystem1 : Subsystem  RequirementInfo="{'linktype_rmi_doors' '0000a538 (/E-STEER Core/SubSystem Specifications/Application Functions/SF031A Current Reasonableness Diagnostic)' '#SF031A_138' 'true' 'REQ:  SF031A_138' '' } %GIDa_f93e60f2_5067_48f8_a504_00b9b916d1ca"  TreatAsAtomicUnit=on
  If1 : If  RequirementInfo={} %GIDa_14f49605_63f5_43ac_82c2_758f32acbb1d  IfExpression=u1 == 1
  LimDyn_f32 : NxtrLim/LimDyn_f32  RequirementInfo="{'linktype_rmi_doors' '0000a538 (/E-STEER Core/SubSystem Specifications/Application Functions/SF031A Current Reasonableness Diagnostic)' '#SF031A_146' 'true' 'REQ:  SF031A_146' '' } %GIDa_0d712b77_cc20_44f6_b13f_a1a074f15ed8"
  Math Function : Math  RequirementInfo="{'linktype_rmi_doors' '0000a538 (/E-STEER Core/SubSystem Specifications/Application Functions/SF031A Current Reasonableness Diagnostic)' '#SF031A_159' 'true' 'REQ:  SF031A_159' '' } %GIDa_183a4a3b_5d73_4dd0_97de_20a93d8f9b51"  Operator=square  SaturateOnIntegerOverflow=on
  Math Function1 : Math  RequirementInfo="{'linktype_rmi_doors' '0000a538 (/E-STEER Core/SubSystem Specifications/Application Functions/SF031A Current Reasonableness Diagnostic)' '#SF031A_159' 'true' 'REQ:  SF031A_159' '' } %GIDa_25f2455a_c604_4627_be44_613260e9a782"  Operator=square  SaturateOnIntegerOverflow=on
  Merge : Merge
  Product1 : Product  Inputs=3  RndMeth=Zero
  Product14 : Product  RequirementInfo={} %GIDa_87342d8c_9b61_49fc_a4ca_73817f7af217  RndMeth=Zero
  Product2 : Product  RequirementInfo="{'linktype_rmi_doors' '0000a538 (/E-STEER Core/SubSystem Specifications/Application Functions/SF031A Current Reasonableness Diagnostic)' '#SF031A_111' 'true' 'REQ:  SF031A_111' '' } %GIDa_4001a904_8b28_4791_a438_cc810bade18a"  RndMeth=Zero
  Product5 : Product  RequirementInfo="{'linktype_rmi_doors' '0000a538 (/E-STEER Core/SubSystem Specifications/Application Functions/SF031A Current Reasonableness Diagnostic)' '#SF031A_111' 'true' 'REQ:  SF031A_111' '' } %GIDa_f872ab5e_db27_4240_800d_09dd8148292e"  RndMeth=Zero
  Product6 : Product  RequirementInfo="{'linktype_rmi_doors' '0000a538 (/E-STEER Core/SubSystem Specifications/Application Functions/SF031A Current Reasonableness Diagnostic)' '#SF031A_111' 'true' 'REQ:  SF031A_111' '' } %GIDa_ea983e5c_7626_4bd2_8a0d_f60d955dfe0b"  RndMeth=Zero
  Product7 : Product  RequirementInfo="{'linktype_rmi_doors' '0000a538 (/E-STEER Core/SubSystem Specifications/Application Functions/SF031A Current Reasonableness Diagnostic)' '#SF031A_112' 'true' 'REQ:  SF031A_112' '' } %GIDa_1423d2cc_06c6_4ed8_b8c8_ed43ba0e97ec"  RndMeth=Zero
  Product8 : Product  RequirementInfo="{'linktype_rmi_doors' '0000a538 (/E-STEER Core/SubSystem Specifications/Application Functions/SF031A Current Reasonableness Diagnostic)' '#SF031A_112' 'true' 'REQ:  SF031A_112' '' } %GIDa_b5567423_cfcd_4b18_aae9_4eaa6c525fba"  RndMeth=Zero
  Sin_f32 : NxtrMath/Sin_f32  RequirementInfo="{'linktype_rmi_doors' '0000a538 (/E-STEER Core/SubSystem Specifications/Application Functions/SF031A Current Reasonableness Diagnostic)' '#SF031A_111' 'true' 'REQ:  SF031A_111' '' } %GIDa_bdff5aca_dc74_4833_a007_3dfd0e2c7343"  SFunctionSpec=single y1 = Sin_f32(single u1)
      settings: AttributesFormatString=%<MaskType>
  Sqrt1 : Sqrt  RequirementInfo="{'linktype_rmi_doors' '0000a538 (/E-STEER Core/SubSystem Specifications/Application Functions/SF031A Current Reasonableness Diagnostic)' '#SF031A_159' 'true' 'REQ:  SF031A_159' '' } %GIDa_7b575b54_589c_4a7c_8391_2b6da3c6d19b"  SaturateOnIntegerOverflow=on
  Tustin Filter1 : Subsystem  RequirementInfo="{'linktype_rmi_doors' '0000a538 (/E-STEER Core/SubSystem Specifications/Application Functions/SF031A Current Reasonableness Diagnostic)' '#SF031A_157' 'true' 'REQ:  SF031A_157' '' } %GIDa_26003aeb_1c4a_4af7_8ca0_b3fb96974c09"
  Tustin Filter2 : Subsystem  RequirementInfo="{'linktype_rmi_doors' '0000a538 (/E-STEER Core/SubSystem Specifications/Application Functions/SF031A Current Reasonableness Diagnostic)' '#SF031A_158' 'true' 'REQ:  SF031A_158' '' } %GIDa_e3bec294_13ae_41fc_afa7_8a5f54bde2f7"
  wires:
  Add/1 -> [Term1], Data Store Write1/1
  SysMotTqCmdSca/1 -> CurrReasbn Diagnostic/3(SysMotTqCmdSca)
  MotTqCmdLimrMin/1 -> CurrReasbn Diagnostic/2(TqLimMin)
  MotVltgQaxFild/1 -> Add/1
  MotVltgQaxFfStat/1 -> Add/2
  MotVltgDaxFild/1 -> Add1/1
  MotVltgDaxFfStat/1 -> Add1/2
  Add1/1 -> Data Store Write2/1, [Term2]
  [MotVltgDiagFild] -> CurrReasbn Diagnostic/1(MotVltgDiagFild)
  Sqrt1/1 -> [MotVltgDiagFild], Data Store Write5/1
  Product8/1 -> Add3/2
  Product6/1 -> Add2/2
  Add3/1 -> Tustin Filter2/1(Input)
  Constant3/1 -> Product2/2
  MotAgElec/1 -> Product2/1
  Sin_f32/1 -> Product5/2, Product7/2
  [Term1] -> Product5/1
  Product5/1 -> Add2/1
  [Term2] -> Product6/1
  Cos_f32/1 -> Product8/2, Product6/2
  [Term2] -> Product7/1
  Product7/1 -> Add3/1
  [Term1] -> Product8/1
  Product2/1 -> Cos_f32/1, Sin_f32/1
  Tustin Filter2/1(Output) -> Data Store Write4/1, Math Function1/1
  Tustin Filter1/1(Output) -> Math Function/1, Data Store Write3/1
  Math Function/1 -> Add4/1
  Add4/1 -> Sqrt1/1
  Math Function1/1 -> Add4/2
  [FrqRadPerSec] -> Tustin Filter2/2(Cutoff)
  If Action Subsystem/1(Out1) -> Merge/1
  If Action Subsystem1/1(Out1) -> Merge/2
  If1/1 -> If Action Subsystem/Action
  If1/2 -> If Action Subsystem1/Action
  [FrqRadPerSec] -> Tustin Filter1/2(Cutoff)
  Add2/1 -> Tustin Filter1/1(Input)
  Constant/1 -> LimDyn_f32/3
  Constant1/1 -> LimDyn_f32/2
  Product14/1 -> Product1/3
  Constant10/1 -> Product1/2
  Constant2/1 -> Product14/1
  Constant9/1 -> Product14/2
  MotVelMrf/1 -> Abs/1
  Product1/1 -> [FrqRadPerSec]
  LimDyn_f32/1 -> Product1/1
  Merge/1 -> LimDyn_f32/1, Data Store Write6/1
  Constant4/1 -> If1/1
  Abs/1 -> If Action Subsystem1/1(In1), If Action Subsystem/1(In1)

== system SF031A_CurrReasbnDiagc/CurrReasbnDiagc/CurrReasbnDiagcInit1/CopyRight2 ==

== system SF031A_CurrReasbnDiagc/CurrReasbnDiagc/CurrReasbnDiagcInit2/CopyRight2 ==

== system SF031A_CurrReasbnDiagc/CurrReasbnDiagc/CurrReasbnDiagcPer1/CopyRight2 ==

== system SF031A_CurrReasbnDiagc/CurrReasbnDiagc/CurrReasbnDiagcPer1/If Action Subsystem ==
  In1 : Inport
  Action Port : ActionPort  ActionType=then
  CopyRight2 : Subsystem  Description=|  mask(Copyright Information){none=on}
      | Copyright info block.                                               
      |                                                                     
      | Place copyright information at the top of every subsystem in design.
      mask prompts: none "No parameters"
      mask help: Place copyright information at the top of every subsystem in design.
      mask Display:
      | NxtrConf = 'Nexteer Confidential';
      | 
      | sys = bdroot; %handle for the current model ("system")
      | first = get_param(sys,'Created');
      | if(isempty(first))
      |     first = datestr(now,'yyyy');
      | else
      |     first = first(end-3:end);  %year is last four digits
      | end
      | 
      | last = get_param(sys,'LastModifiedDate');
      | if isempty(last)
      |     last = datestr(now,'yyyy');
      | else
      |     last = last(end-3:end);
      | end
      | 
      | if strcmp(first,last)
      |     fprintf('%s -- Copyright %s Nexteer',NxtrConf,first)
      | else
      |     fprintf('%s -- %s%s- %s Nexteer',NxtrConf,char(169),first,last)
      | end
  Out1 : Outport
  wires:
  In1/1 -> Out1/1

== system SF031A_CurrReasbnDiagc/CurrReasbnDiagc/CurrReasbnDiagcPer1/If Action Subsystem1 ==
  In1 : Inport
  Action Port : ActionPort  ActionType=else
  CopyRight2 : Subsystem  Description=|  mask(Copyright Information){none=on}
      | Copyright info block.                                               
      |                                                                     
      | Place copyright information at the top of every subsystem in design.
      mask prompts: none "No parameters"
      mask help: Place copyright information at the top of every subsystem in design.
      mask Display:
      | NxtrConf = 'Nexteer Confidential';
      | 
      | sys = bdroot; %handle for the current model ("system")
      | first = get_param(sys,'Created');
      | if(isempty(first))
      |     first = datestr(now,'yyyy');
      | else
      |     first = first(end-3:end);  %year is last four digits
      | end
      | 
      | last = get_param(sys,'LastModifiedDate');
      | if isempty(last)
      |     last = datestr(now,'yyyy');
      | else
      |     last = last(end-3:end);
      | end
      | 
      | if strcmp(first,last)
      |     fprintf('%s -- Copyright %s Nexteer',NxtrConf,first)
      | else
      |     fprintf('%s -- %s%s- %s Nexteer',NxtrConf,char(169),first,last)
      | end
  Out1 : Outport
  wires:
  In1/1 -> Out1/1

== system SF031A_CurrReasbnDiagc/CurrReasbnDiagc/CurrReasbnDiagcPer1/If Action Subsystem2 ==
  In1 : Inport
  Action Port : ActionPort  ActionType=then
  CopyRight2 : Subsystem  Description=|  mask(Copyright Information){none=on}
      | Copyright info block.                                               
      |                                                                     
      | Place copyright information at the top of every subsystem in design.
      mask prompts: none "No parameters"
      mask help: Place copyright information at the top of every subsystem in design.
      mask Display:
      | NxtrConf = 'Nexteer Confidential';
      | 
      | sys = bdroot; %handle for the current model ("system")
      | first = get_param(sys,'Created');
      | if(isempty(first))
      |     first = datestr(now,'yyyy');
      | else
      |     first = first(end-3:end);  %year is last four digits
      | end
      | 
      | last = get_param(sys,'LastModifiedDate');
      | if isempty(last)
      |     last = datestr(now,'yyyy');
      | else
      |     last = last(end-3:end);
      | end
      | 
      | if strcmp(first,last)
      |     fprintf('%s -- Copyright %s Nexteer',NxtrConf,first)
      | else
      |     fprintf('%s -- %s%s- %s Nexteer',NxtrConf,char(169),first,last)
      | end
  Out1 : Outport
  wires:
  In1/1 -> Out1/1

== system SF031A_CurrReasbnDiagc/CurrReasbnDiagc/CurrReasbnDiagcPer1/If Action Subsystem3 ==
  In1 : Inport
  Action Port : ActionPort  ActionType=else
  CopyRight2 : Subsystem  Description=|  mask(Copyright Information){none=on}
      | Copyright info block.                                               
      |                                                                     
      | Place copyright information at the top of every subsystem in design.
      mask prompts: none "No parameters"
      mask help: Place copyright information at the top of every subsystem in design.
      mask Display:
      | NxtrConf = 'Nexteer Confidential';
      | 
      | sys = bdroot; %handle for the current model ("system")
      | first = get_param(sys,'Created');
      | if(isempty(first))
      |     first = datestr(now,'yyyy');
      | else
      |     first = first(end-3:end);  %year is last four digits
      | end
      | 
      | last = get_param(sys,'LastModifiedDate');
      | if isempty(last)
      |     last = datestr(now,'yyyy');
      | else
      |     last = last(end-3:end);
      | end
      | 
      | if strcmp(first,last)
      |     fprintf('%s -- Copyright %s Nexteer',NxtrConf,first)
      | else
      |     fprintf('%s -- %s%s- %s Nexteer',NxtrConf,char(169),first,last)
      | end
  Out1 : Outport
  wires:
  In1/1 -> Out1/1

== system SF031A_CurrReasbnDiagc/CurrReasbnDiagc/CurrReasbnDiagcPer2/CopyRight2 ==
